simulink model "PR1_var15"  (R2020b)
settings: Solver=FixedStepAuto  StartTime=0.0  StopTime=10  FixedStep=0.001  RelTol=1e-3
settings Model: Creator=SIA  LastModifiedBy=SIA

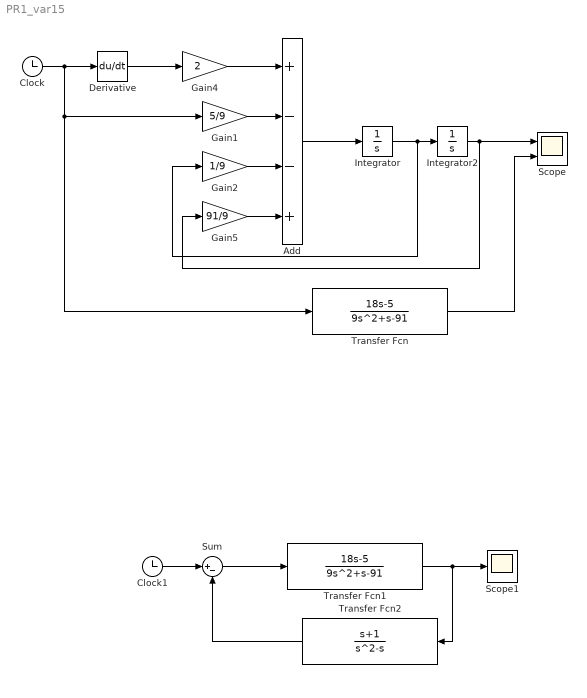
== system PR1_var15 ==
  Add : Sum  Inputs=+--+
  Clock : Clock
  Clock1 : Clock
  Derivative : Derivative
  Gain1 : Gain  Gain=5/9
  Gain2 : Gain  Gain=1/9
  Gain4 : Gain  Gain=2
  Gain5 : Gain  Gain=91/9
  Integrator : Integrator
  Integrator2 : Integrator
  Scope : Scope  NumInputPorts=2
  Scope1 : Scope
  Sum : Sum  Inputs=|+-
  Transfer Fcn : TransferFcn  Numerator=[18 -5]  Denominator=[9 1 -91]
  Transfer Fcn1 : TransferFcn  Numerator=[18 -5]  Denominator=[9 1 -91]
  Transfer Fcn2 : TransferFcn  Numerator=[1 1]  Denominator=[1 -1 0]
  wires:
  Gain4/1 -> Add/1
  Transfer Fcn/1 -> Scope/2
  Derivative/1 -> Gain4/1
  Integrator2/1 -> Gain5/1, Scope/1
  Gain1/1 -> Add/2
  Transfer Fcn2/1 -> Sum/2
  Clock/1 -> Derivative/1, Transfer Fcn/1, Gain1/1
  Clock1/1 -> Sum/1
  Gain2/1 -> Add/3
  Add/1 -> Integrator/1
  Transfer Fcn1/1 -> Scope1/1, Transfer Fcn2/1
  Sum/1 -> Transfer Fcn1/1
  Gain5/1 -> Add/4
  Integrator/1 -> Gain2/1, Integrator2/1
